simulink model "TestFrottementsNew"  (R2024b)
settings: Solver=VariableStepAuto  StartTime=0.0  StopTime=10.0  RelTol=1e-3
undefined symbols (not defined in the file): Kv, RegimeTq, TempsTq, TorqueLosesTest, TorqueLosesTimeTest, Vcyl
settings Model: Creator=a030141  LastModifiedBy=ramse
settings DebuggingCC: UnderspecifiedInitializationDetection=Classic  MergeDetectMultiDrivingBlocksExec=none
settings ModelReferenceCC: PropagateSignalLabelsOutOfModel=off

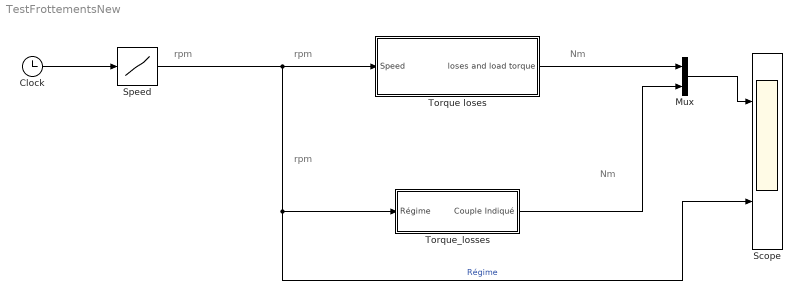
== system TestFrottementsNew ==
  note: Nm
  note: rpm
  note: rpm
  note: rpm
  note: Nm
  " Torque loses" : Subsystem
  Clock : Clock
  Mux : Mux  Inputs=2
  Scope : Scope  NumInputPorts=2
  Speed : Lookup  InputValues=TempsTq  Table=RegimeTq
  Torque_losses : Subsystem
  wires:
  Clock/1 -> Speed/1
  Speed/1 -> Scope/2, Torque_losses/1(Régime), " Torque loses"/1(Speed)  "Régime"
  Mux/1 -> Scope/1
  " Torque loses"/1(loses and load torque) -> Mux/1
  Torque_losses/1(Couple Indiqué) -> Mux/2

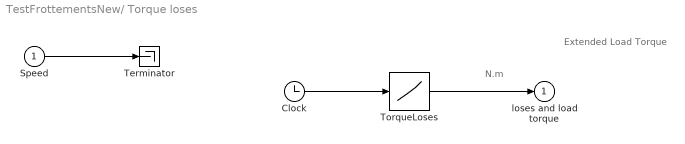
== system TestFrottementsNew/ Torque loses ==
  note: N.m
  note: Extended Load Torque
  Speed : Inport
  Clock : Clock
  Terminator : Terminator
  TorqueLoses : Lookup  InputValues=TorqueLosesTimeTest  Table=TorqueLosesTest
  loses and load torque : Outport
  wires:
  Clock/1 -> TorqueLoses/1
  TorqueLoses/1 -> loses and load torque/1
  Speed/1 -> Terminator/1

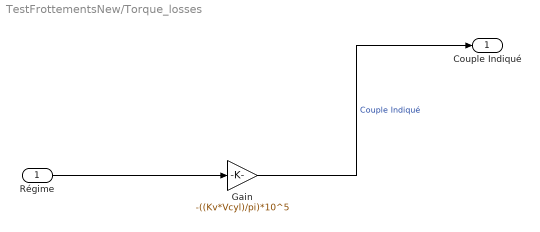
== system TestFrottementsNew/Torque_losses ==
  Régime : Inport
  Gain : Gain  Gain=-((Kv*Vcyl)/pi)*10^5
  Couple Indiqué : Outport
  wires:
  Régime/1 -> Gain/1
  Gain/1 -> Couple Indiqué/1  "Couple Indiqué"
